simulink model "flightControlSystem"  (R2023a)
settings: Solver=ode3  StartTime=0  StopTime=TFinal  FixedStep=Ts  RelTol=1e-3  EnableMultiTasking=on
undefined symbols (not defined in the file): afterTime, codertarget, COG_X, COG_Y, Controller, corner_step, degree_range1, degree_range2, degree_range3, DiscIntNeverNeededParam, Discrete, epsilon, Estimator, g, Gamma, gray, init, modi_PI, num_threshold, over_step, prev_degree_range, prev_degree_range2, Q, R, radius, radius2, ROI_Size, rotation_degree, rotation_degree2, Sensors, straight_step, strel, Time, Ts, tuning1, tuning11, tuning2, var_acc_angle_N, var_bias_gyr_N, var_gyro_p_N, Vehicle
libraries: simulink x41, slpidlib x4, ctrlSharedLib x4, visiontransforms x4, visiontextngfix x4, sharedtransform x3, visionanalysis x3, simulink_need_slupdate x1, parrotlib x1, visionmorphops x1
(part 4 of 4)

== matlab function flightControlSystem/Image Processing System/corner detection subsystem1/straight line detector/center_line maker ==
  data: center_lines output; flag_corner output; Theta input; Rho input; cnt input; label input; error output
function [center_lines, flag_corner, error] = fcn(Theta, Rho, cnt, label)
    % cnt에 따라 케이스 나누기
    % cnt = 0일 때 오류 => error = 1;
    % cnt = 1일 때 오류 => error = 1;
    % cnt = 2일 때 flag_corner=0 그리고 center_lines 1개 뽑기
    % cnt = 3일 때 flag_corner=1 그리고 center_lines 1개 뽑기(동일한 theta값 외에 한 직선은 무시하는 알고리즘 필요)
    % cnt = 4일 때 flag_corner=1 그리고 center_lines 2개 뽑기
    center_lines = zeros(2,2);
    flag_corner = 0;
    error = 0;
    if cnt == 0 || cnt == 1
        error = 1;
    elseif cnt == 2
        idx1 = find(label==1,1);
        rho1 = Rho(idx1(1));
        theta1 = Theta(idx1(1));
        idx2 = find(label==2,1);
        rho2 = Rho(idx2(1));
        theta2 = Theta(idx2(1));
        if min(abs(theta1 - theta2),180-abs(theta1 - theta2)) <deg2rad(10)
            center_lines(1,1) = (rho1+rho2)/2;
            center_lines(1,2) = (theta1+theta2)/2;
        else
            error = 1;
        end
    elseif cnt == 3
        flag_corner = 1;
        idx1 = find(label==1,1);
        rho1 = Rho(idx1(1));
        theta1 = Theta(idx1(1));
        idx2 = find(label==2,1);
        rho2 = Rho(idx2(1));
        theta2 = Theta(idx2(1));
        idx3 = find(label==3,1);
        rho3 = Rho(idx3(1));
        theta3 = Theta(idx3(1));
        if min(abs(theta1 - theta2),180-abs(theta1 - theta2)) <deg2rad(10)
            center_lines(1,1) = (rho1+rho2)/2;
            center_lines(1,2) = (theta1+theta2)/2;
        elseif min(abs(theta1 - theta3),180-abs(theta1 - theta3)) <deg2rad(10)
            center_lines(1,1) = (rho1+rho3)/2;
            center_lines(1,2) = (theta1+theta3)/2;
        elseif min(abs(theta2 - theta3),180-abs(theta2 - theta3)) <deg2rad(10)
            center_lines(1,1) = (rho2+rho3)/2;
            center_lines(1,2) = (theta2+theta3)/2;
        else
            error = 1;
        end
    elseif cnt == 4
        flag_corner = 1;
        idx1 = find(label==1,1);
        rho1 = Rho(idx1(1));
        theta1 = Theta(idx1(1));
        idx2 = find(label==2,1);
        rho2 = Rho(idx2(1));
        theta2 = Theta(idx2(1));
        idx3 = find(label==3,1);
        rho3 = Rho(idx3(1));
        theta3 = Theta(idx3(1));
        idx4 = find(label==4,1);
        rho4 = Rho(idx4(1));
        theta4 = Theta(idx4(1));
        if min(abs(theta1 - theta2),180-abs(theta1 - theta2)) <deg2rad(10)
            center_lines(1,1) = (rho1+rho2)/2;
            center_lines(1,2) = (theta1+theta2)/2;
            
            center_lines(2,1) = (rho3+rho4)/2;
            center_lines(2,2) = (theta3+theta4)/2;
        elseif min(abs(theta1 - theta3),180-abs(theta1 - theta3)) <deg2rad(10)
            center_lines(1,1) = (rho1+rho3)/2;
            center_lines(1,2) = (theta1+theta3)/2;
        
            center_lines(2,1) = (rho2+rho4)/2;
            center_lines(2,2) = (theta2+theta4)/2;
        elseif min(abs(theta1 - theta4),180-abs(theta1 - theta4)) <deg2rad(10)
            center_lines(1,1) = (rho1+rho4)/2;
            center_lines(1,2) = (theta1+theta4)/2;
            
            center_lines(2,1) = (rho2+rho3)/2;
            center_lines(2,2) = (theta2+theta3)/2;
        else
            error = 1;
        end
    end

== matlab function flightControlSystem/Image Processing System/Result of previous work for backup/delete tail ==
  data: dots input; sorting_ref input; COG_X parameter; COG_Y parameter; MAP output; cutting_dots output
function [MAP, cutting_dots] = fcn(dots, sorting_ref, COG_X, COG_Y)


num_dots = size(dots,1);
cutting_dots = zeros(num_dots,2);
degree_reange = 90;

% sorting_ref의 두 번째 값을 이전값으로 사용,(일단은 이렇게. 수정이 필요할 수도.)
if sorting_ref == 0
    prev_dx = 0;
    prev_dy = 0;
end
prev_dx = sorting_ref(2,1);
prev_dy = sorting_ref(2,2);



prev_deg = mod(atan2(prev_dy,prev_dx)+pi,2*pi); % 이전 진행 방향 + pi

idx = 1;
MAP=zeros(120,160);
for i=1:num_dots
    if abs( mod(atan2(dots(i,2)-COG_Y, COG_X-dots(i,1)),2*pi)  -  prev_deg) > degree_reange*pi/180  &&  dots(i,1) ~= 0
        cutting_dots(idx,1) = dots(i,1);
        cutting_dots(idx,2) = dots(i,2);
        
        MAP(dots(i,1),dots(i,2))=1;
        idx = idx+1;
    end
end

== matlab function flightControlSystem/Image Processing System/Subsystem1/MATLAB Function ==
  data: prev_points input; weightMeanPoint output
function weightMeanPoint = fcn(prev_points)

k1 = 1.6;
k2 = 0.9;
k3 = 0.5;


weightMeanPoint = ( k1*prev_points(1,:) + k2*prev_points(2,:) + k3*prev_points(3,:) ) / 3;

== matlab function flightControlSystem/Image Processing System/corner detection subsystem1/straight line detector/corner_finder ==
  data: center_Pts input; corner output; cnt input
function corner = fcn(center_Pts,cnt)
corner = zeros(1,2);
if cnt==4
    % Define the points on the first line
    P1 = [center_Pts(1,1) center_Pts(1,2)];
    P2 = [center_Pts(1,3) center_Pts(1,4)];
    % Define the points on the second line
    Q1 = [center_Pts(2,1) center_Pts(2,2)];
    Q2 = [center_Pts(2,3) center_Pts(2,4)];
    if P2(1) - P1(1) == 0 % The first line is vertical
        % Calculate the slope and y-intercept of the second line
        slope_Q = (Q2(2) - Q1(2)) / (Q2(1) - Q1(1));
        y_intercept2 = Q1(2) - slope_Q * Q1(1);

        % Calculate the intersection point
        x_intersect = P1(1);
        y_intersect = slope_Q * x_intersect + y_intercept2;
    elseif Q2(1) - Q1(1) == 0 % The second line is vertical
        % Calculate the slope and y-intercept of the first line
        slope_P = (P2(2) - P1(2)) / (P2(1) - P1(1));
        y_intercept1 = P1(2) - slope_P * P1(1);

        % Calculate the intersection point
        x_intersect = Q1(1);
        y_intersect = slope_P * x_intersect + y_intercept1;
    else % Both lines are not vertical
        % Calculate the slope and y-intercept of each line
        slope_P = (P2(2) - P1(2)) / (P2(1) - P1(1));
        y_intercept1 = P1(2) - slope_P * P1(1);
        slope_Q = (Q2(2) - Q1(2)) / (Q2(1) - Q1(1));
        y_intercept2 = Q1(2) - slope_Q * Q1(1);

        % Calculate the intersection point
        x_intersect = (y_intercept2 - y_intercept1) / (slope_P - slope_Q);
        y_intersect = slope_P * x_intersect + y_intercept1;
    end
    % Output the intersection point
    corner = [y_intersect, x_intersect];
end

== matlab function flightControlSystem/Image Processing System/corner detection subsystem1/straight line detector/hough trans ==
  data: edge_image input; Theta output; Rho output; cnt output; label output
function [Theta,Rho,cnt,label] = fcn(edge_image)
    [H,T,R] = hough(edge_image);
    P = houghpeaks(H,4,'Threshold',0.3*max(H(:)),'NHoodSize',[19 19]);
    Theta = zeros(4,1);
    Rho = zeros(4,1);
    n = size(P,1);
    for i=1:n
        Rho(i) = R(P(i,1));
        Theta(i) = deg2rad(T(P(i,2)));
    end
    cnt = 0; %서로 다른 라인의 개수
    label = zeros(4,1); %같은 라인끼리 묶는 집합
    for i = 1:n
        if label(i)==0
            cnt = cnt + 1;
            label(i) = cnt;
            if i<n
                for j = i+1:n
                    if label(j) == 0 && abs(Rho(i)-Rho(j))<10 && min(180-abs(Theta(i)-Theta(j)),abs(Theta(i)-Theta(j)))<deg2rad(10)
                            label(j) = cnt;
                    end
                end
            end
        end
    end

== matlab function flightControlSystem/Image Processing System/MATLAB Function1 ==
  data: bin_image input; prev_ref input; y output; ref1 input; ref2 input; corner input; flag_corner input; COG_X parameter; COG_Y parameter
function y = fcn(bin_image, prev_ref,ref1,ref2,corner, flag_corner,COG_X, COG_Y)
y = zeros(120,160,3);

for i=1:120
    for j=1:160
        if bin_image(i,j)
            y(i,j,:) = [255 255 255];
        end
    end
end

% C = round([corner(1);corner(2)]);% blue
% P = round([prev_ref(1,1);prev_ref(1,2)]);% yellow
R1 = round([COG_X-ref1(1);ref1(2)+COG_Y]);% red
R2 = round([COG_X-ref2(1);ref2(2)+COG_Y]);% purple
% if flag_corner
%     for i = C(1)-1:C(1)+1
%         for j=C(2)-1:C(2)+1
%             if i>=1 && i<=120 && j>=1 && j<=160
%             y(i,j,:)=[0 0 255]; 
%             end
%         end
%     end
% end
% for i = P(1)-1:P(1)+1
%     for j=P(2)-1:P(2)+1
%         if i>=1 && i<=120 && j>=1 && j<=160
%             y(i,j,:)=[200 200 0]; 
%         end
%     end
% end
for i = R1(1)-1:R1(1)+1
    for j=R1(2)-1:R1(2)+1
        if i>=1 && i<=120 && j>=1 && j<=160
            y(i,j,:)=[255 0 0]; 
        end
    end
end
for i = R2(1)-1:R2(1)+1
    for j=R2(2)-1:R2(2)+1
        if i>=1 && i<=120 && j>=1 && j<=160
            y(i,j,:)=[200 0 200]; 
        end
    end
end

% Drone pos
for i = COG_X-1:COG_X+1
    for j=COG_Y-1:COG_Y+1
        if i>=1 && i<=120 && j>=1 && j<=160 && mod(i+j,2)==0
            y(i,j,:)=[0 0 255]; 
        end
    end
end

== matlab function flightControlSystem/Control System/Path Planning/MATLAB Function ==
  data: u input; y output; clock input
function y = fcn(u, clock)
persistent cnt
persistent first
persistent st_check
if isempty(cnt)
    cnt=clock;
    st_check=0;
    first=0;
end
if u==0 && clock>3.5
    if(clock-st_check<.6)
        y=1;
        return
    else
        y=u;
        return
    end
end
if first==1|| clock>3.5
    st_check=clock;
    y=u;
    return;
end
y=1;
if u==0
    cnt=clock;
else
    if clock-cnt>2
        first=1;
    end
end

== matlab function flightControlSystem/Control System/Path Planning/MATLAB Function1 ==
  data: pos input; ref_x output; dp input; ref_y output; over_step input; corner input; tuning1 input; tuning2 input; tuning11 input
function [ref_x,ref_y] = fcn(pos,dp,over_step,corner, tuning1,tuning2,tuning11)

if corner==0
over_step=over_step+1.5;
end

x=pos(1);
y=pos(2);

cl_dx=dp(1,1);
cl_dy=dp(2,1);

fa_dx=dp(1,2);
fa_dy=dp(2,2);

close_x=x+cl_dx;
close_y=y+cl_dy;

far_x=x+fa_dx*over_step;
far_y=y+fa_dy*over_step;

over_dx=far_x-close_x;
over_dy=far_y-close_y;

over_x=far_x+over_dx*over_step;
over_y=far_y+over_dy*over_step;

ref_x=zeros(10,1);
ref_y=zeros(10,1);



persistent the_old_x;
persistent the_old_y;

persistent old_x;
persistent old_y;


if isempty(the_old_x)
    the_old_x=close_x;
    the_old_y=close_y;
    old_x=close_x;
    old_y=close_y;
end



first_dx=(the_old_x-x)/2;
first_dy=(the_old_y-y)/2;

second_div=2;
check_dv=0;

second_dx=(old_x-the_old_x)/(second_div+check_dv);
second_dy=(old_y-the_old_y)/(second_div+check_dv);

third_dx=(close_x-old_x)/3;
third_dy=(close_x-old_x)/3;

forth_dx=(over_x-close_x)/3;
forth_dy=(over_y-close_y)/3;

ref_x(1)=x+first_dx;
ref_y(1)=y+first_dy;
ref_x(2)=ref_x(1)+first_dx;
ref_y(2)=ref_y(1)+first_dy;


for i=3-check_dv:4
    ref_x(i,1)=ref_x(i-1,1)+second_dx;
    ref_y(i,1)=ref_y(i-1,1)+second_dy;
end

for i=5:7
    ref_x(i,1)=ref_x(i-1,1)+third_dx;
    ref_y(i,1)=ref_y(i-1,1)+third_dy;
end
for i=8:10
    ref_x(i,1)=ref_x(i-1,1)+forth_dx;
    ref_y(i,1)=ref_y(i-1,1)+forth_dy;
end

if (sqrt(first_dx^2+first_dy^2)>=0.06)
    ref_x(1)=old_x;
    ref_y(1)=old_y;


    third_dx=(close_x-old_x)/tuning1;
    third_dy=(close_x-old_x)/tuning1;

    forth_dx=(over_x-close_x)/tuning2;
    forth_dy=(over_y-close_y)/tuning2;

    
    for i=2:tuning11
        ref_x(i,1)=ref_x(i-1,1)+third_dx;
        ref_y(i,1)=ref_y(i-1,1)+third_dy;
    end
    for i=(tuning11+1):10
        ref_x(i,1)=ref_x(i-1,1)+forth_dx;
        ref_y(i,1)=ref_y(i-1,1)+forth_dy;
    end

end

% persistent temp_x
% persistent temp_y
% 
% if(isempty(temp_x))
%     temp_x=close_x;
%     temp_y=close_y;
% end
% if clock<2
%     first_dx=(temp_x-x)/10;
%     first_dy=(temp_y-y)/10;
% 
%     ref_x(1)=x+first_dx;
%     ref_y(1)=y+first_dy;
% 
%     for i=2:10
%         ref_x(i)=ref_x(i-1)+first_dx;
%         ref_y(i)=ref_y(i-1)+first_dy;
% 
%     end
% end

the_old_x=old_x;
the_old_y=old_y;
old_x=close_x;
old_y=close_y;
end

== matlab function flightControlSystem/Control System/Path Planning/mpc/MATLAB Function ==
  data: u input; y output
function y = fcn(u)
y=0;

if(mod(u,0.2)==0)
   y=1; 
end

== matlab function flightControlSystem/Image Processing System/delete_segment2 ==
  data: seg_image output; bin_image input; COG_X parameter; COG_Y parameter
function seg_image   = delete_segment(bin_image,COG_X, COG_Y)

% dots = zeros(19200 , 2);
% idx = 1;
% for i = 1:120
%    for j = 1:160
%       if bin_image(i, j) == 1
%          dots(idx,1) = i;
%          dots(idx,2) = j;
%          idx = idx + 1;
%       end
%    end
% end
% 
% center = [COG_X, COG_Y];
% k = dsearchn(dots ,center);
% x = dots(k,1);
% y = dots(k,2);
% 

L = bwlabel(bin_image,8);
label = L(COG_X, COG_Y);
if label==0
    label = 1;
end
seg_image = L==label;

== matlab function flightControlSystem/Image Processing System/corner detection subsystem/corner_detector/hough trans ==
  data: edge_image input; flag_corner output; param_Hough parameter
function flag_corner  = fcn(edge_image,param_Hough)
    [H,T,R] = hough(edge_image);
    P = houghpeaks(H,4,'Threshold',param_Hough*max(H(:)),'NHoodSize',[19 19]);
    Theta = zeros(4,1);
    Rho = zeros(4,1);
    n = size(P,1);
    for i=1:n
        Rho(i) = R(P(i,1));
        Theta(i) = deg2rad(T(P(i,2)));
    end
    cnt = 0; %서로 다른 라인의 개수
    label = zeros(4,1); %같은 라인끼리 묶는 집합
    for i = 1:n
        if label(i)==0
            cnt = cnt + 1;
            label(i) = cnt;
            if i<n
                for j = i+1:n
                    if label(j) == 0 && abs(Rho(i)-Rho(j))<10 && min(180-abs(Theta(i)-Theta(j)),abs(Theta(i)-Theta(j)))<deg2rad(10)
                            label(j) = cnt;
                    end
                end
            end
        end
    end
    if cnt>=3
        flag_corner = 1;
    else
        flag_corner = 0;
    end

== matlab function flightControlSystem/Image Processing System/NAN filter/MATLAB Function ==
  data: ref input; y output
function y = fcn(ref)

if (ref(1,1) == 60 && ref(1,2) == -80 ) ||  isnan(ref(1,1))
    y = [0,0];
else
    y = ref;
end


% persistent prev_ref1;
% persistent prev_ref2;
% persistent prev_ref3;
% 
% if isempty(prev_ref1)
%     prev_ref1 = zeros(1,2);
% end
% if isempty(prev_ref2)
%     prev_ref2 = zeros(1,2);
% end
% if isempty(prev_ref3)
%     prev_ref3 = zeros(1,2);
% end
% 
% 
% 
% 
% if ref(1,1) == 60 && ref(1,2) == -80
%     if prev_ref2(1,1) == 60 && prev_ref2(1,2) == -80
%         y = prev_ref3;
%     end
%     y = prev_ref2;
% else
%     y = ref;
% end
% 
% prev_ref3 = prev_ref2;
% prev_ref2 = prev_ref1;
% prev_ref1 = ref;

== matlab function flightControlSystem/Image Processing System/MATLAB Function4 ==
  data: bin_image input; y output; ref1 input; ref2 input; COG_X parameter; COG_Y parameter
function y = fcn(bin_image,ref1,ref2,COG_X, COG_Y)
y = zeros(120,160,3);

for i=1:120
    for j=1:160
        if bin_image(i,j)
            y(i,j,:) = [255 255 255];
        end
    end
end

R1 = round([COG_X-ref1(1);ref1(2)+COG_Y]);% red
R2 = round([COG_X-ref2(1);ref2(2)+COG_Y]);% purple
% if flag_corner
%     for i = C(1)-1:C(1)+1
%         for j=C(2)-1:C(2)+1
%             if i>=1 && i<=120 && j>=1 && j<=160
%             y(i,j,:)=[0 0 255]; 
%             end
%         end
%     end
% end
% for i = P(1)-1:P(1)+1
%     for j=P(2)-1:P(2)+1
%         if i>=1 && i<=120 && j>=1 && j<=160
%             y(i,j,:)=[200 200 0]; 
%         end
%     end
% end
if R1(1)>=1 && R1(1)<=120 && R1(2)>=1 && R1(2)<=160
    for i = R1(1)-1:R1(1)+1
        for j=R1(2)-1:R1(2)+1
            if i>=1 && i<=120 && j>=1 && j<=160
                y(i,j,:)=[255 0 0]; 
            end
        end
    end
end
if R2(1)>=1 && R2(1)<=120 && R2(2)>=1 && R2(2)<=160
    for i = R2(1)-1:R2(1)+1
        for j=R2(2)-1:R2(2)+1
            if i>=1 && i<=120 && j>=1 && j<=160
                y(i,j,:)=[200 0 200]; 
            end
        end
    end
end

% Drone pos
for i = COG_X-1:COG_X+1
    for j=COG_Y-1:COG_Y+1
        if i>=1 && i<=120 && j>=1 && j<=160 && mod(i+j,2)==0
            y(i,j,:)=[0 0 255]; 
        end
    end
end

== matlab function flightControlSystem/Image Processing System/MATLAB Function5 ==
  data: u input; R output; G output; B output
function [R,G,B] = fcn(u)
R = u(:,:,1);
G = u(:,:,2);
B = u(:,:,3);

== matlab function flightControlSystem/Image Processing System/corner detection1/delete_segment1 ==
  data: bin_image input; seg_image output; COG_X parameter; COG_Y parameter
function seg_image = delete_segment(bin_image,COG_X, COG_Y)
L = bwlabel(bin_image,8);
label = L(COG_X,COG_Y);
if label==0
    label = 1;
end
seg_image = L==label;

== matlab function flightControlSystem/Image Processing System/corner detection1/straight line detector/center_line maker ==
  data: center_lines output; flag_corner output; Theta input; Rho input; cnt input; label input; error output
function [center_lines, flag_corner, error] = fcn(Theta, Rho, cnt, label)
    % cnt에 따라 케이스 나누기
    % cnt = 0일 때 오류 => error = 1;
    % cnt = 1일 때 오류 => error = 1;
    % cnt = 2일 때 flag_corner=0 그리고 center_lines 1개 뽑기
    % cnt = 3일 때 flag_corner=1 그리고 center_lines 1개 뽑기(동일한 theta값 외에 한 직선은 무시하는 알고리즘 필요)
    % cnt = 4일 때 flag_corner=1 그리고 center_lines 2개 뽑기
    center_lines = zeros(2,2);
    flag_corner = 0;
    error = 0;
    if cnt == 0 || cnt == 1
        error = 1;
    elseif cnt == 2
        idx1 = find(label==1,1);
        rho1 = Rho(idx1(1));
        theta1 = Theta(idx1(1));
        idx2 = find(label==2,1);
        rho2 = Rho(idx2(1));
        theta2 = Theta(idx2(1));
        if min(abs(theta1 - theta2),180-abs(theta1 - theta2)) <deg2rad(10)
            center_lines(1,1) = (rho1+rho2)/2;
            center_lines(1,2) = (theta1+theta2)/2;
        else
            error = 1;
        end
    elseif cnt == 3
        flag_corner = 1;
        idx1 = find(label==1,1);
        rho1 = Rho(idx1(1));
        theta1 = Theta(idx1(1));
        idx2 = find(label==2,1);
        rho2 = Rho(idx2(1));
        theta2 = Theta(idx2(1));
        idx3 = find(label==3,1);
        rho3 = Rho(idx3(1));
        theta3 = Theta(idx3(1));
        if min(abs(theta1 - theta2),180-abs(theta1 - theta2)) <deg2rad(10)
            center_lines(1,1) = (rho1+rho2)/2;
            center_lines(1,2) = (theta1+theta2)/2;
        elseif min(abs(theta1 - theta3),180-abs(theta1 - theta3)) <deg2rad(10)
            center_lines(1,1) = (rho1+rho3)/2;
            center_lines(1,2) = (theta1+theta3)/2;
        elseif min(abs(theta2 - theta3),180-abs(theta2 - theta3)) <deg2rad(10)
            center_lines(1,1) = (rho2+rho3)/2;
            center_lines(1,2) = (theta2+theta3)/2;
        else
            error = 1;
        end
    elseif cnt == 4
        flag_corner = 1;
        idx1 = find(label==1,1);
        rho1 = Rho(idx1(1));
        theta1 = Theta(idx1(1));
        idx2 = find(label==2,1);
        rho2 = Rho(idx2(1));
        theta2 = Theta(idx2(1));
        idx3 = find(label==3,1);
        rho3 = Rho(idx3(1));
        theta3 = Theta(idx3(1));
        idx4 = find(label==4,1);
        rho4 = Rho(idx4(1));
        theta4 = Theta(idx4(1));
        if min(abs(theta1 - theta2),180-abs(theta1 - theta2)) <deg2rad(10)
            center_lines(1,1) = (rho1+rho2)/2;
            center_lines(1,2) = (theta1+theta2)/2;
            
            center_lines(2,1) = (rho3+rho4)/2;
            center_lines(2,2) = (theta3+theta4)/2;
        elseif min(abs(theta1 - theta3),180-abs(theta1 - theta3)) <deg2rad(10)
            center_lines(1,1) = (rho1+rho3)/2;
            center_lines(1,2) = (theta1+theta3)/2;
        
            center_lines(2,1) = (rho2+rho4)/2;
            center_lines(2,2) = (theta2+theta4)/2;
        elseif min(abs(theta1 - theta4),180-abs(theta1 - theta4)) <deg2rad(10)
            center_lines(1,1) = (rho1+rho4)/2;
            center_lines(1,2) = (theta1+theta4)/2;
            
            center_lines(2,1) = (rho2+rho3)/2;
            center_lines(2,2) = (theta2+theta3)/2;
        else
            error = 1;
        end
    end

== matlab function flightControlSystem/Image Processing System/corner detection1/straight line detector/corner_finder ==
  data: center_Pts input; corner output; cnt input
function corner = fcn(center_Pts,cnt)
corner = zeros(1,2);
if cnt==4
    % Define the points on the first line
    P1 = [center_Pts(1,1) center_Pts(1,2)];
    P2 = [center_Pts(1,3) center_Pts(1,4)];
    % Define the points on the second line
    Q1 = [center_Pts(2,1) center_Pts(2,2)];
    Q2 = [center_Pts(2,3) center_Pts(2,4)];
    if P2(1) - P1(1) == 0 % The first line is vertical
        % Calculate the slope and y-intercept of the second line
        slope_Q = (Q2(2) - Q1(2)) / (Q2(1) - Q1(1));
        y_intercept2 = Q1(2) - slope_Q * Q1(1);

        % Calculate the intersection point
        x_intersect = P1(1);
        y_intersect = slope_Q * x_intersect + y_intercept2;
    elseif Q2(1) - Q1(1) == 0 % The second line is vertical
        % Calculate the slope and y-intercept of the first line
        slope_P = (P2(2) - P1(2)) / (P2(1) - P1(1));
        y_intercept1 = P1(2) - slope_P * P1(1);

        % Calculate the intersection point
        x_intersect = Q1(1);
        y_intersect = slope_P * x_intersect + y_intercept1;
    else % Both lines are not vertical
        % Calculate the slope and y-intercept of each line
        slope_P = (P2(2) - P1(2)) / (P2(1) - P1(1));
        y_intercept1 = P1(2) - slope_P * P1(1);
        slope_Q = (Q2(2) - Q1(2)) / (Q2(1) - Q1(1));
        y_intercept2 = Q1(2) - slope_Q * Q1(1);

        % Calculate the intersection point
        x_intersect = (y_intercept2 - y_intercept1) / (slope_P - slope_Q);
        y_intersect = slope_P * x_intersect + y_intercept1;
    end
    % Output the intersection point
    corner = [y_intersect, x_intersect];
end

== matlab function flightControlSystem/Image Processing System/corner detection1/straight line detector/hough trans of center lines ==
  data: center_lines input; Theta output; Rho output
function [Theta,Rho] = fcn(center_lines)
    Theta = center_lines(:,2);
    Rho = center_lines(:,1);

== matlab function flightControlSystem/Image Processing System/corner detection1/straight line detector/hough trans ==
  data: edge_image input; Theta output; Rho output; cnt output; label output
function [Theta,Rho,cnt,label] = fcn(edge_image)
    [H,T,R] = hough(edge_image);
    P = houghpeaks(H,4,'Threshold',0.3*max(H(:)),'NHoodSize',[19 19]);
    Theta = zeros(4,1);
    Rho = zeros(4,1);
    n = size(P,1);
    for i=1:n
        Rho(i) = R(P(i,1));
        Theta(i) = deg2rad(T(P(i,2)));
    end
    cnt = 0; %서로 다른 라인의 개수
    label = zeros(4,1); %같은 라인끼리 묶는 집합
    for i = 1:n
        if label(i)==0
            cnt = cnt + 1;
            label(i) = cnt;
            if i<n
                for j = i+1:n
                    if label(j) == 0 && abs(Rho(i)-Rho(j))<10 && min(180-abs(Theta(i)-Theta(j)),abs(Theta(i)-Theta(j)))<deg2rad(10)
                            label(j) = cnt;
                    end
                end
            end
        end
    end

== matlab function flightControlSystem/Control System/Path Planning/dot_follow ==
  data: data input; u input; final_pos output; end_flag output
function [final_pos,end_flag] = fcn(data, u)
final_pos=zeros(3,1);
final_pos(1)=data(1)+u(1,1);
final_pos(2)=data(2)+u(2,1);
final_pos(3)=-1.3;
end_flag=0;

if(abs(u(1))<0.05&&abs(u(2))<0.05)
    final_pos(3)=0;
    end_flag=1;
end

== matlab function flightControlSystem/Control System/Path Planning/MATLAB Function2 ==
  data: flag input; clock input; pose output; pos input
function pose = fcn(flag,clock, pos)
persistent x
persistent y
persistent tempf
persistent cnt
persistent land
pose=zeros(3,1);
if isempty(x)
    x=0;
    y=0;
    tempf=0;
    cnt=0;
    land=0;
end



if tempf==0 || (flag==1 && clock<2)
    pose=pos;
elseif tempf==1 && clock>2
    pose(1)=x;
    pose(2)=y;
    if (abs(pos(1)-pose(1))>0.001 && abs(pos(2)-pose(2))>0.001)&&land==0
        pose(3)=-1.3;
        land=0;
        return
    end
    pose(3)=0;
    land=1;
    return
end
if flag==1 &&x==0 &&clock>2
    cnt=cnt+1;
    if cnt>400
        x=pos(1);
        y=pos(2);
        tempf=1;
    end
end

== matlab function flightControlSystem/Image Processing System/corner detection subsystem1/straight line detector/hough trans of center lines ==
  data: center_lines input; Theta output; Rho output
function [Theta,Rho] = fcn(center_lines)
    Theta = center_lines(:,2);
    Rho = center_lines(:,1);

== matlab function flightControlSystem/Image Processing System/NAN filter/MATLAB Function2 ==
  data: ref1 input; y output; ref2 input
function y = fcn(ref1,ref2)

if (ref1(1,1) == 0 && ref1(1,2) == 0 ) ||  isnan(ref2(1,1))
    y = [0,0];
else
    y = ref2;
end
